simulink model "PoliArd_PID_2015a"  (R2015a)
settings: Solver=ode3  StartTime=0.0  StopTime=inf  FixedStep=0.001  RelTol=1e-3
values from neighbouring files (symbols this model uses):
  b = 0.025    [Main_PoliArd_PID.m]
undefined symbols (not defined in the file or in its folder): cx, cy, KIy, KPy
libraries: PoliArd x10, simulink x2, simulink_extras x2
settings Model: CovHtmlReporting=off  ExtModeTrigDuration=2  Creator=User  LastModifiedBy=User
settings OptimizationCC: LifeSpan=1
settings DebuggingCC: UnderspecifiedInitializationDetection=Classic  MergeDetectMultiDrivingBlocksExec=none
settings HardwareCC: ProdLargestAtomicInteger=Long  ProdLargestAtomicFloat=Double  ProdEndianess=LittleEndian  ProdHWDeviceType=ARM Compatible->ARM Cortex
settings RTWCC: SystemTargetFile=realtime.tlc  GenerateMakefile=off  TemplateMakefile=realtime.tmf  Description=Run on Target Hardware  RTWVerbose=off
settings ERTTargetCC: CombineOutputUpdateFcns=off  ExtModeTransport=3  ExtModeMexFile=ext_serial_win32_comm_rtt  ExtModeMexArgs=0 1 9600  InlinedParameterPlacement=Hierarchical  ERTSrcFileBannerTemplate=realtime_code_template.cgt  ERTHdrFileBannerTemplate=realtime_code_template.cgt  ERTDataSrcFileTemplate=realtime_code_template.cgt  ERTDataHdrFileTemplate=realtime_code_template.cgt  ERTCustomFileTemplate=realtime_file_process.tlc

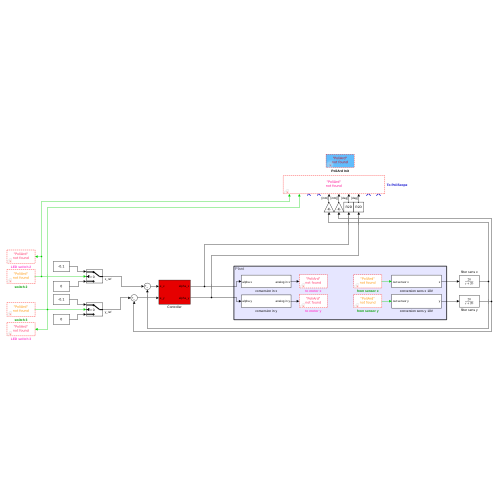
[thumbnail: Simulink's stored preview of the top-level diagram]
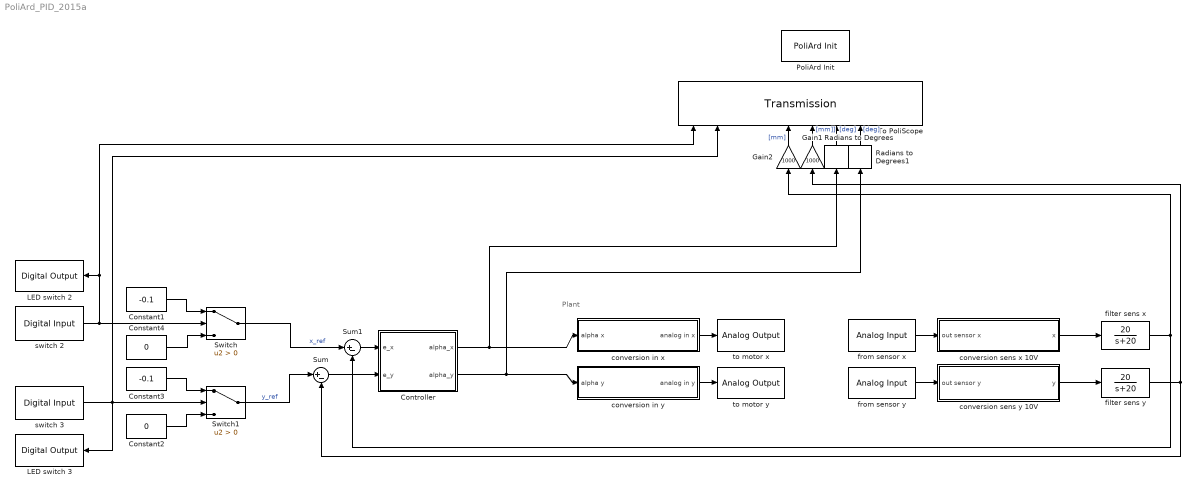
== system PoliArd_PID_2015a ==
  note: Plant
  Constant1 : Constant  Value=-0.1
  Constant2 : Constant  Value=0
  Constant3 : Constant  Value=-0.1
  Constant4 : Constant  Value=0
  Controller : Subsystem
  Gain1 : Gain  Gain=1000
  Gain2 : Gain  Gain=1000
  "LED switch 2 " : PoliArd/Digital Output  DO_pin=1
  "LED switch 3 " : PoliArd/Digital Output  DO_pin=2
  PoliArd Init : PoliArd/PoliArd Init
  Radians to Degrees : simulink_extras/Transformations/Radians to Degrees
  Radians to Degrees1 : simulink_extras/Transformations/Radians to Degrees
  Sum : Sum  Inputs=|+-
  Sum1 : Sum  Inputs=|+-
  Switch : Switch  Criteria=u2 > Threshold
  Switch1 : Switch  Criteria=u2 > Threshold
  To PoliScope : PoliArd/Transmission  sample_freq=1000  sig_to_send=6
  conversion in x : Subsystem
  conversion in y : Subsystem
  conversion sens x 10V : Subsystem
  conversion sens y 10V : Subsystem
  filter sens x : TransferFcn  Numerator=[20]  Denominator=[1 20]
  filter sens y : TransferFcn  Numerator=[20]  Denominator=[1 20]
  from sensor x : PoliArd/Analog Input  AIpin_mask=4  AIsample=-1
  from sensor y : PoliArd/Analog Input  AIpin_mask=3  AIsample=-1
  switch 2 : PoliArd/Digital Input  DI_pin=2  DIsample=-1
  switch 3 : PoliArd/Digital Input  DI_pin=3  DIsample=-1
  to motor x : PoliArd/Analog Output  DAC_pin_mask=1
  to motor y : PoliArd/Analog Output  DAC_pin_mask=2
  wires:
  filter sens y/1 -> Sum/2, Gain1/1
  filter sens x/1 -> Sum1/2, Gain2/1
  Gain1/1 -> To PoliScope/6  "[mm]]"
  Gain2/1 -> To PoliScope/5  "[mm]"
  from sensor x/1 -> conversion sens x 10V/1(out sensor x)
  from sensor y/1 -> conversion sens y 10V/1(out sensor y)
  conversion in x/1(analog in x) -> to motor x/1
  conversion in y/1(analog in y) -> to motor y/1
  Controller/2(alpha_y) -> conversion in y/1(alpha y), Radians to Degrees1/1
  Controller/1(alpha_x) -> Radians to Degrees/1, conversion in x/1(alpha x)
  conversion sens x 10V/1(x) -> filter sens x/1
  conversion sens y 10V/1(y) -> filter sens y/1
  Constant1/1 -> Switch/1
  Switch/1 -> Sum1/1  "x_ref"
  Constant3/1 -> Switch1/1
  Constant2/1 -> Switch1/3
  Switch1/1 -> Sum/1  "y_ref"
  Sum/1 -> Controller/2(e_y)
  Sum1/1 -> Controller/1(e_x)
  switch 3/1 -> Switch1/2, "LED switch 3 "/1, To PoliScope/2
  Constant4/1 -> Switch/3
  switch 2/1 -> Switch/2, To PoliScope/1, "LED switch 2 "/1
  Radians to Degrees/1 -> To PoliScope/7  "[deg]"
  Radians to Degrees1/1 -> To PoliScope/8  "[deg]"

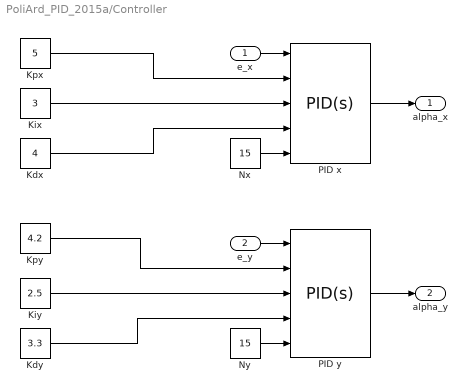
== system PoliArd_PID_2015a/Controller ==
  e_x : Inport
  e_y : Inport  Port=2
  Kdx : Constant  Value=4
  "Kdy " : Constant  Value=3.3
  Kix : Constant  Value=3
  Kiy : Constant  Value=2.5
  Kpx : Constant  Value=5
  Kpy : Constant  Value=4.2
  Nx : Constant  Value=15
  Ny : Constant  Value=15
  PID x : simulink/Continuous/PID Controller  Controller=PID  TimeDomain=Continuous-time  SampleTime=-1  IntegratorMethod=Forward Euler  FilterMethod=Forward Euler  Form=Parallel  UseFilter=on  ControllerParametersSource=external  P=5  I=2  D=6  N=30  InitialConditionSource=internal  InitialConditionForIntegrator=0  InitialConditionForFilter=0  ExternalReset=none  LimitOutput=on  UpperSaturationLimit=deg2rad(75)  LowerSaturationLimit=deg2rad(-75)  LinearizeAsGain=on  AntiWindupMode=back-calculation  Kb=0.8  TrackingMode=off  Kt=1  PParamMin=[]  PParamMax=[]  IParamMin=[]  IParamMax=[]  DParamMin=[]  DParamMax=[]  NParamMin=[]  NParamMax=[]  KbParamMin=[]  KbParamMax=[]  KtParamMin=[]  KtParamMax=[]  POutMin=[]  POutMax=[]  IOutMin=[]  IOutMax=[]  DOutMin=[]  DOutMax=[]  NOutMin=[]  NOutMax=[]  KbOutMin=[]  KbOutMax=[]  KtOutMin=[]  KtOutMax=[]  IntegratorOutMin=[]  IntegratorOutMax=[]  FilterOutMin=[]  FilterOutMax=[]  SumOutMin=[]  SumOutMax=[]  SumI1OutMin=[]  SumI1OutMax=[]  SumI2OutMin=[]  SumI2OutMax=[]  SumI3OutMin=[]  SumI3OutMax=[]  SumDOutMin=[]  SumDOutMax=[]  SaturationOutMin=[]  SaturationOutMax=[]  IntegratorContinuousStateAttributes=''  IntegratorStateMustResolveToSignalObject=off  IntegratorRTWStateStorageClass=Auto  FilterContinuousStateAttributes=''  FilterStateMustResolveToSignalObject=off  FilterRTWStateStorageClass=Auto  DifferentiatorICPrevScaledInput=0  DifferentiatorOutMin=[]  DifferentiatorOutMax=[]
  PID y : simulink/Continuous/PID Controller  Controller=PID  TimeDomain=Continuous-time  SampleTime=-1  IntegratorMethod=Forward Euler  FilterMethod=Forward Euler  Form=Parallel  UseFilter=on  ControllerParametersSource=external  P=KPy  I=KIy  D=-0.189219016325203  N=1.72044274974478  InitialConditionSource=internal  InitialConditionForIntegrator=0  InitialConditionForFilter=0  ExternalReset=none  LimitOutput=on  UpperSaturationLimit=deg2rad(30)  LowerSaturationLimit=deg2rad(-30)  LinearizeAsGain=on  AntiWindupMode=back-calculation  Kb=0.8  TrackingMode=off  Kt=1  PParamMin=[]  PParamMax=[]  IParamMin=[]  IParamMax=[]  DParamMin=[]  DParamMax=[]  NParamMin=[]  NParamMax=[]  KbParamMin=[]  KbParamMax=[]  KtParamMin=[]  KtParamMax=[]  POutMin=[]  POutMax=[]  IOutMin=[]  IOutMax=[]  DOutMin=[]  DOutMax=[]  NOutMin=[]  NOutMax=[]  KbOutMin=[]  KbOutMax=[]  KtOutMin=[]  KtOutMax=[]  IntegratorOutMin=[]  IntegratorOutMax=[]  FilterOutMin=[]  FilterOutMax=[]  SumOutMin=[]  SumOutMax=[]  SumI1OutMin=[]  SumI1OutMax=[]  SumI2OutMin=[]  SumI2OutMax=[]  SumI3OutMin=[]  SumI3OutMax=[]  SumDOutMin=[]  SumDOutMax=[]  SaturationOutMin=[]  SaturationOutMax=[]  IntegratorContinuousStateAttributes=''  IntegratorStateMustResolveToSignalObject=off  IntegratorRTWStateStorageClass=Auto  FilterContinuousStateAttributes=''  FilterStateMustResolveToSignalObject=off  FilterRTWStateStorageClass=Auto  DifferentiatorICPrevScaledInput=0  DifferentiatorOutMin=[]  DifferentiatorOutMax=[]
  alpha_x : Outport
  alpha_y : Outport  Port=2
  wires:
  PID y/1 -> alpha_y/1
  PID x/1 -> alpha_x/1
  e_x/1 -> PID x/1
  e_y/1 -> PID y/1
  Nx/1 -> PID x/5
  Ny/1 -> PID y/5
  Kix/1 -> PID x/3
  Kpy/1 -> PID y/2
  "Kdy "/1 -> PID y/4
  Kpx/1 -> PID x/2
  Kdx/1 -> PID x/4
  Kiy/1 -> PID y/3

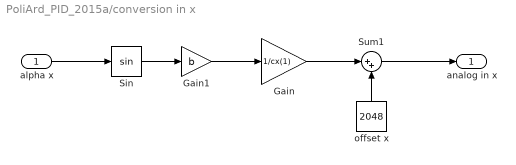
== system PoliArd_PID_2015a/conversion in x ==
  alpha x : Inport
  Gain : Gain  Gain=1/cx(1)
  Gain1 : Gain  Gain=b
  Sin : Trigonometry
  Sum1 : Sum  Inputs=|++
  offset x : Constant  Value=2048
  analog in x : Outport
  wires:
  Sin/1 -> Gain1/1
  Gain1/1 -> Gain/1
  Gain/1 -> Sum1/1
  Sum1/1 -> analog in x/1
  offset x/1 -> Sum1/2
  alpha x/1 -> Sin/1

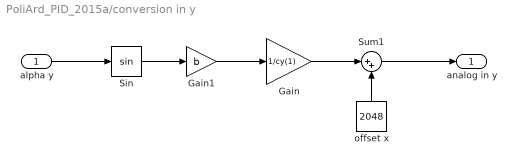
== system PoliArd_PID_2015a/conversion in y ==
  alpha y : Inport
  Gain : Gain  Gain=1/cy(1)
  Gain1 : Gain  Gain=b
  Sin : Trigonometry
  Sum1 : Sum  Inputs=|++
  offset x : Constant  Value=2048
  analog in y : Outport
  wires:
  alpha y/1 -> Sin/1
  offset x/1 -> Sum1/2
  Sum1/1 -> analog in y/1
  Gain/1 -> Sum1/1
  Gain1/1 -> Gain/1
  Sin/1 -> Gain1/1

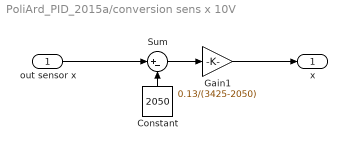
== system PoliArd_PID_2015a/conversion sens x 10V ==
  out sensor x : Inport
  Constant : Constant  Value=2050
  Gain1 : Gain  Gain=0.13/(3425-2050)
  Sum : Sum  Inputs=|+-
  x : Outport
  wires:
  Constant/1 -> Sum/2
  Sum/1 -> Gain1/1
  out sensor x/1 -> Sum/1
  Gain1/1 -> x/1

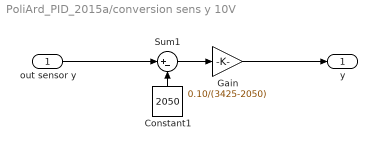
== system PoliArd_PID_2015a/conversion sens y 10V ==
  out sensor y : Inport
  Constant1 : Constant  Value=2050
  Gain : Gain  Gain=0.10/(3425-2050)
  Sum1 : Sum  Inputs=|+-
  y : Outport
  wires:
  out sensor y/1 -> Sum1/1
  Sum1/1 -> Gain/1
  Constant1/1 -> Sum1/2
  Gain/1 -> y/1
